simulink model "QgcServerSim_v2022b"  (R2022b)
settings: Solver=FixedStepAuto  StartTime=0.0  StopTime=inf  FixedStep=1e-2  MaxStep=1e-2  RelTol=1e-3
model workspace (MATLAB code in the model file):
  | % function MacroDef()
  | 
  | % //Omni端数据的state定义
  | % #define OMNI_SEND_STATE_ERROR -100
  | global OMNI_SEND_STATE_ERROR
  | OMNI_SEND_STATE_ERROR = (-100);
  | % #define OMNI_SEND_STATE_EMPTY 0
  | global OMNI_SEND_STATE_EMPTY
  | OMNI_SEND_STATE_EMPTY = (0);
  | % #define OMNI_SEND_STATE_HEARTBEAT 10
  | global OMNI_SEND_STATE_HEARTBEAT
  | OMNI_SEND_STATE_HEARTBEAT = (10);
  | % #define OMNI_SEND_STATE_SYN 20
  | global OMNI_SEND_STATE_SYN
  | OMNI_SEND_STATE_SYN = (20);
  | % #define OMNI_SEND_STATE_ONLY_NOTE 30
  | global OMNI_SEND_STATE_ONLY_NOTE
  | OMNI_SEND_STATE_ONLY_NOTE = (30);
  | % #define OMNI_SEND_STATE_CURRENT_CORE 100
  | global OMNI_SEND_STATE_CURRENT_CORE
  | OMNI_SEND_STATE_CURRENT_CORE = (100);
  | % #define OMNI_SEND_STATE_LAST_CORE 101
  | global OMNI_SEND_STATE_LAST_CORE
  | OMNI_SEND_STATE_LAST_CORE = (101);
  | % #define OMNI_SEND_STATE_CURRENT_POSE 200
  | global OMNI_SEND_STATE_CURRENT_POSE
  | OMNI_SEND_STATE_CURRENT_POSE = (200);
  | % #define OMNI_SEND_STATE_LAST_POSE 201
  | global OMNI_SEND_STATE_LAST_POSE
  | OMNI_SEND_STATE_LAST_POSE = (201);
  | % #define OMNI_SEND_STATE_CURRENT_FORCE 300
  | global OMNI_SEND_STATE_CURRENT_FORCE
  | OMNI_SEND_STATE_CURRENT_FORCE = (300);
  | % #define OMNI_SEND_STATE_LAST_FORCE 301
  | global OMNI_SEND_STATE_LAST_FORCE
  | OMNI_SEND_STATE_LAST_FORCE = (301);
  | % #define OMNI_RCV_STATE_EMPTY 1000
  | global OMNI_RCV_STATE_EMPTY
  | OMNI_RCV_STATE_EMPTY = (1000);
  | % #define OMNI_RCV_STATE_HEARTBEAT 1010
  | global OMNI_RCV_STATE_HEARTBEAT
  | OMNI_RCV_STATE_HEARTBEAT = (1010);
  | % #define OMNI_RCV_STATE_TRIGGER 1020
  | global OMNI_RCV_STATE_TRIGGER
  | OMNI_RCV_STATE_TRIGGER = (1020);
  | % #define OMNI_RCV_STATE_CONFIG 1100
  | global OMNI_RCV_STATE_CONFIG
  | OMNI_RCV_STATE_CONFIG = (1100);
  | % #define OMNI_RCV_STATE_FORCE 1300
  | global OMNI_RCV_STATE_FORCE
  | OMNI_RCV_STATE_FORCE = (1300);
  | % #define OMNI_RCV_STATE_TORQUE 1301
  | global OMNI_RCV_STATE_TORQUE
  | OMNI_RCV_STATE_TORQUE = (1301);
  | 
  | % end
libraries: sldrtlib x2, slrealtimeiplib x2
settings Model: Creator=WDDSC  LastModifiedBy=WDDSC

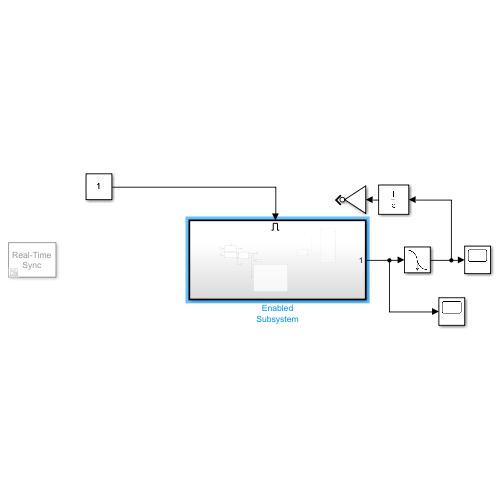
[thumbnail: Simulink's stored preview of the top-level diagram]
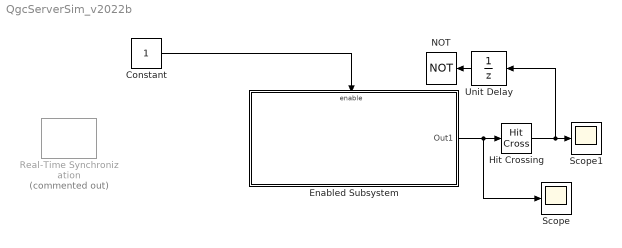
== system QgcServerSim_v2022b ==
  Constant : Constant
  Enabled Subsystem : Subsystem  TreatAsAtomicUnit=on
  Hit Crossing : HitCross  HitCrossingOffset=0.5  HitCrossingDirection=falling
  NOT : Logic  Operator=NOT  IconShape=distinctive  AllPortsSameDT=off  OutDataTypeStr=boolean
  Real-Time Synchronization : sldrtlib/Real-Time Synchronization  Commented=on  SampleTime=1e-2  MaxMissedTicks=10  ShowMissedTicks=off  YieldWhenWaiting=off
  Scope : Scope
  Scope1 : Scope
  Unit Delay : UnitDelay  SampleTime=-1  HasFrameUpgradeWarning=on
  wires:
  Enabled Subsystem/1(Out1) -> Scope/1, Hit Crossing/1
  Hit Crossing/1 -> Scope1/1, Unit Delay/1
  Unit Delay/1 -> NOT/1
  Constant/1 -> Enabled Subsystem/Enable

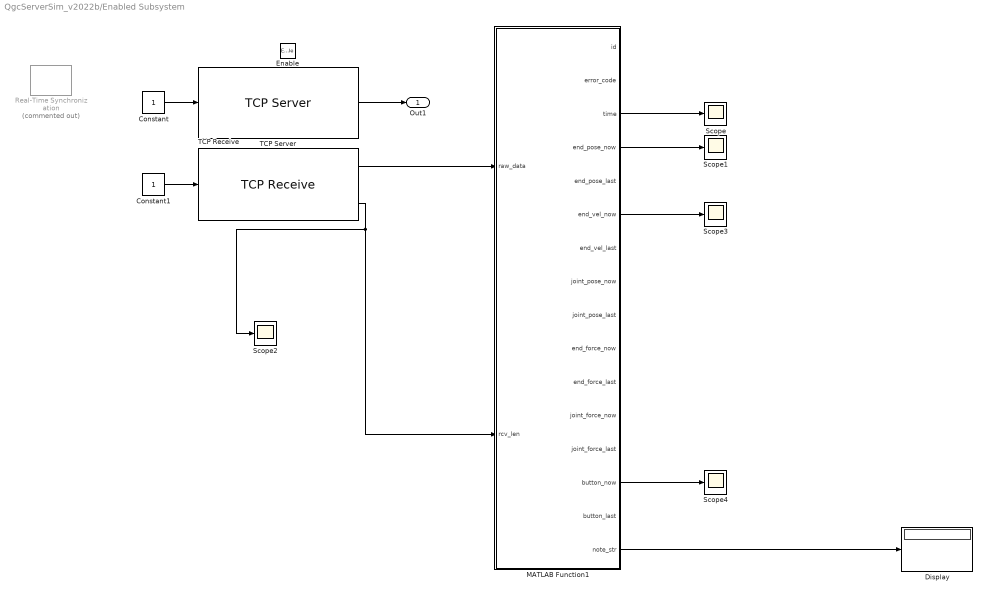
== system QgcServerSim_v2022b/Enabled Subsystem ==
  Enable : EnablePort  StatesWhenEnabling=reset
  Constant : Constant
  Constant1 : Constant
  Display : Display
  MATLAB Function1 : MATLAB Function  TreatAsAtomicUnit=on
  Real-Time Synchronization : sldrtlib/Real-Time Synchronization  Commented=on  SampleTime=1e-2  MaxMissedTicks=inf  ShowMissedTicks=off  YieldWhenWaiting=off
  Scope{,1..4} (5 alike) : Scope
  TCP Receive : slrealtimeiplib/TCP Receive  socketAddPortVal=Server: 127.0.0.1:10301  rcvWidth=40960  sampleTime=-1
  TCP Server : slrealtimeiplib/TCP Server  Priority=-1  useHostTargetConn=off  serverAddress=127.0.0.1  serverPort=10301
  Out1 : Outport
  wires:
  TCP Server/1 -> Out1/1
  Constant/1 -> TCP Server/1
  TCP Receive/1 -> MATLAB Function1/1(raw_data)
  Constant1/1 -> TCP Receive/1
  TCP Receive/2 -> Scope2/1, MATLAB Function1/2(rcv_len)
  MATLAB Function1/4(end_pose_now) -> Scope1/1
  MATLAB Function1/16(note_str) -> Display/1
  MATLAB Function1/3(time) -> Scope/1
  MATLAB Function1/6(end_vel_now) -> Scope3/1
  MATLAB Function1/14(button_now) -> Scope4/1

== matlab function QgcServerSim_v2022b/Enabled Subsystem/MATLAB Function1 ==
  data: id output double size=1; error_code output size=1; time output size=1; end_pose_now output; end_pose_last output; end_vel_now output; end_vel_last output; joint_pose_now output; joint_pose_last output; end_force_now output; end_force_last output; joint_force_now output; joint_force_last output; button_now output; button_last output; note_str output; raw_data input; rcv_len input
% function [trunc_data, id, state, error_code, time] = GrabMsg(raw_data, rcv_len)
% function [error_code, ...
%     end_position, button] = GrabMsg(raw_data, rcv_len)
function [id, error_code, time, ...
    end_pose_now, end_pose_last, ...
    end_vel_now, end_vel_last, ...
    joint_pose_now, joint_pose_last, ...
    end_force_now, end_force_last, ...
    joint_force_now, joint_force_last, ...
    button_now, button_last, ...
    note_str] = GrabMsg(raw_data, rcv_len)

%% 读空数据后，截取一帧

%初始化输出
id = -1;
%state = nan;
error_code = nan;
time = -1;
[end_pose_now, end_pose_last, ...
end_vel_now, end_vel_last, ...
joint_pose_now, joint_pose_last, ...
end_force_now, end_force_last, ...
joint_force_now, joint_force_last] = deal(nan(6,1));
[button_now, button_last] = deal(nan);
note_str = "";

omni_status = getEmptyStatus();

%若接受的数据长度正常（256的倍数），开始处理
if rcv_len <= 0
    error_code = -1;
elseif mod(rcv_len,256) ~= 0
    error_code = -2;
else
    error_code = 0; %只有err=0才代表接受数据成功
    % 遍历所有数据帧，尽量不漏消息
    for iframe = 1 : rcv_len/256
        trunc_data = raw_data((iframe-1)*256+1 : iframe*256);
        tmp = double(typecast(uint8(trunc_data(5:8)), 'int32'));
        id = max([id, tmp(1)]);
        %state = double(typecast(uint8(trunc_data(9:12)), 'int32'));
        tmp = max(double(typecast(uint8(trunc_data(13:16)), 'int32')));
        error_code = max([error_code, tmp(1)]);
        tmp = double(typecast(uint8(trunc_data(17:24)), 'int64'));
        time = max([time, tmp(1)]);
        omni_status = solveStatus(trunc_data, omni_status);
    end
end

%输出量赋值

end_pose_now(1:3) = omni_status.end_position_now(1:3);
end_pose_now(4:6) = omni_status.joint_angles_now(1:3);
end_pose_last(1:3) = omni_status.end_position_last(1:3);
end_pose_last(4:6) = omni_status.joint_angles_last(1:3);

end_vel_now(1:3) = omni_status.end_velocity_now(1:3);
end_vel_now(4:6) = omni_status.gimbal_velocity_now(1:3);
end_vel_last(1:3) = omni_status.end_velocity_last(1:3);
end_vel_last(4:6) = omni_status.gimbal_velocity_last(1:3);

joint_pose_now(1:3) = omni_status.joint_angles_now(1:3);
joint_pose_now(4:6) = omni_status.gimbal_angles_now(1:3);
joint_pose_last(1:3) = omni_status.joint_angles_last(1:3);
joint_pose_last(4:6) = omni_status.gimbal_angles_last(1:3);

end_force_now(1:3) = omni_status.end_force_now(1:3);
end_force_now(4:6) = omni_status.end_torque_now(1:3);
end_force_last(1:3) = omni_status.end_force_last(1:3);
end_force_last(4:6) = omni_status.end_torque_last(1:3);

joint_force_now(1:3) = omni_status.joint_torque_now(1:3);
joint_force_now(4:6) = omni_status.gimbal_torque_now(1:3);
joint_force_last(1:3) = omni_status.joint_torque_last(1:3);
joint_force_last(4:6) = omni_status.gimbal_torque_last(1:3);

button_now = omni_status.button_now(1);
button_last = omni_status.button_last(1);

note_str = omni_status.note_str;
